simulink model "sim_cascade"  (R2020b)
settings: Solver=ode1  StartTime=0.0  StopTime=30  FixedStep=0.01  RelTol=1e-3
undefined symbols (not defined in the file): kd_o, ki_o, kp_i, kp_o
settings Model: Creator=ONLY-GOD  LastModifiedBy=ONLY-GOD

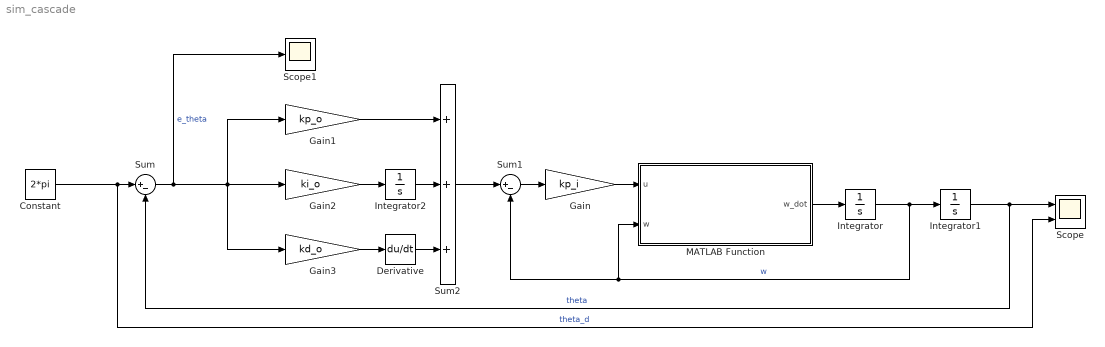
== system sim_cascade ==
  Constant : Constant  Value=2*pi
  Derivative : Derivative
  Gain : Gain  Gain=kp_i
  Gain1 : Gain  Gain=kp_o
  Gain2 : Gain  Gain=ki_o
  Gain3 : Gain  Gain=kd_o
  Integrator : Integrator
  Integrator1 : Integrator
  Integrator2 : Integrator
  MATLAB Function : MATLAB Function  TreatAsAtomicUnit=on
  Scope : Scope  NumInputPorts=2
  Scope1 : Scope
  Sum : Sum  Inputs=|+-
  Sum1 : Sum  Inputs=|+-
  Sum2 : Sum  Inputs=+++
  wires:
  MATLAB Function/1(w_dot) -> Integrator/1
  Integrator/1 -> Integrator1/1, Sum1/2, MATLAB Function/2(w)  "w"
  Gain/1 -> MATLAB Function/1(u)
  Sum1/1 -> Gain/1
  Gain2/1 -> Integrator2/1
  Gain1/1 -> Sum2/1
  Gain3/1 -> Derivative/1
  Sum2/1 -> Sum1/1
  Sum/1 -> Scope1/1, Gain2/1, Gain3/1, Gain1/1  "e_theta"
  Integrator1/1 -> Sum/2, Scope/1  "theta"
  Constant/1 -> Scope/2, Sum/1  "theta_d"
  Derivative/1 -> Sum2/3
  Integrator2/1 -> Sum2/2

== matlab function sim_cascade/MATLAB Function ==
  data: u input; w_dot output; w input
function w_dot = model(u,w)
a = 27.65;
b = 17.35;
c = 5.63;

w_dot = -a*w+b*u;
